simulink model "Simulink_Observation_5"  (R2020b)
settings: Solver=VariableStepAuto  StartTime=0.0  StopTime=0  RelTol=1e-3
libraries: dspvision x2
settings Model: Creator=Mohit Akhouri  LastModifiedBy=Mohit Akhouri

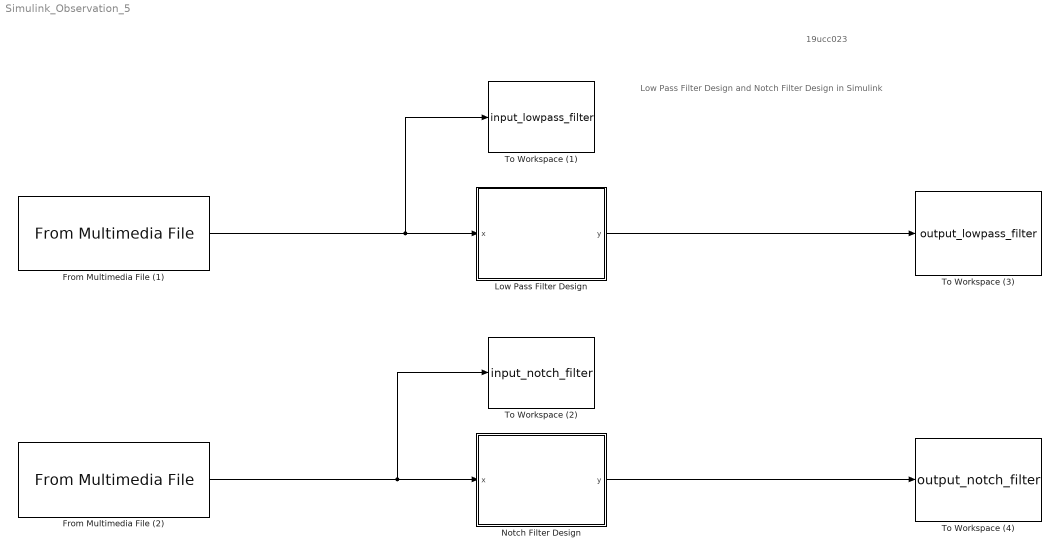
== system Simulink_Observation_5 ==
  note: Low Pass Filter Design and Notch Filter Design in Simulink
  note: 19ucc023
  From Multimedia File (1) : dspvision/From Multimedia File  inputFilename=C:\Users\Mohit Akhouri\Desktop\DSP_LAB_EXP_9\inputwithhissgreaterthanpiby2.wav  readRange=[1 Inf]  loop=on  numPlays=inf  outputStreams=Audio only  videoDataType=single  audioDataType=double  inheritSampleTime=on  userDefinedSampleTime=1/30  noAudioOutput=off  isIntensityVideo=off  fourcc=RGB  colorVideoFormat=Separate color signals  outputEOF=off  dataOrg=Column-major  audioFrameSize=1262848  computeAudioFrameSize=off  outSamplingMode=Sample based
  From Multimedia File (2) : dspvision/From Multimedia File  inputFilename=C:\Users\Mohit Akhouri\Desktop\DSP_LAB_EXP_9\inputwithhissmadelaptop.wav  readRange=[1 Inf]  loop=on  numPlays=inf  outputStreams=Audio only  videoDataType=single  audioDataType=double  inheritSampleTime=on  userDefinedSampleTime=1/30  noAudioOutput=off  isIntensityVideo=off  fourcc=RGB  colorVideoFormat=Separate color signals  outputEOF=off  dataOrg=Column-major  audioFrameSize=1262848  computeAudioFrameSize=off  outSamplingMode=Sample based
  Low Pass Filter Design : MATLAB Function  TreatAsAtomicUnit=on
  Notch Filter Design : MATLAB Function  TreatAsAtomicUnit=on
  To Workspace (1) : ToWorkspace  VariableName=input_lowpass_filter  SaveFormat=Timeseries  SampleTime=-1
  To Workspace (2) : ToWorkspace  VariableName=input_notch_filter  SaveFormat=Timeseries  SampleTime=-1
  To Workspace (3) : ToWorkspace  VariableName=output_lowpass_filter  SaveFormat=Timeseries  SampleTime=-1
  To Workspace (4) : ToWorkspace  VariableName=output_notch_filter  SaveFormat=Timeseries  SampleTime=-1
  wires:
  From Multimedia File (2)/1 -> To Workspace (2)/1, Notch Filter Design/1(x)
  Notch Filter Design/1(y) -> To Workspace (4)/1
  From Multimedia File (1)/1 -> To Workspace (1)/1, Low Pass Filter Design/1(x)
  Low Pass Filter Design/1(y) -> To Workspace (3)/1

== matlab function Simulink_Observation_5/Notch Filter Design ==
  data: x input; y output
function y = fcn(x)
hn = [1 -2*cos(pi/2) 1]; % Filter impulse response for NOTCH FILTER
y = conv(x,hn); % convolution of distorted signal x[n] and impulse response of NOTCH FILTER h[n]

== matlab function Simulink_Observation_5/Low Pass Filter Design ==
  data: x input; y output
function y = fcn(x)

x = x'; % Taking the transpose to convert from Nx1 to 1xN for easy multiplication later on
y = complex(zeros(1,length(x)));
x_length = length(x); % Finding length of audio signal x[n]

samples = 256; % variable to store the sample number for partition of audio file
hw = ones(1,256); % ideal low pass filter impulse response

% making the 66th and 192th sample number = 0
hw(66) = 0;
hw(192) = 0;

% main loop algorithm for dividing the audio file into chunks and
% individually applying fft on each chunk and multiplying with filter
% impulse response to get the smoothened version of audio signal
for i=1:samples:x_length
    x_sampled = x(i:i+255); % taking 256 samples chunk
    x_sampled_fft = fft(x_sampled,256); % taking DFT of the 256 samples
    yw = x_sampled_fft .* hw; % filtering process takes place
    y(i:i+255) = ifft(yw); % rewriting the original audio file with smoothened version of audio
end
